simulink model "Op_Space_Grav_Comp"  (R2020b)
settings: Solver=VariableStepAuto  StartTime=0.0  StopTime=10  RelTol=1e-3
values from neighbouring files (symbols this model uses):
  G = myRobot.G_Lagrangian    [hw9_main.m]
  Ja = Ja(1:3,:)    [hw9_main.m]
  Kd = diag([25,15,15])    [hw9_main.m]
  Kp = diag([28,22,20])    [hw9_main.m]
  xd = [0.3; 0.3; 0.3]    [hw9_main.m]
settings Model: Creator=nicol  LastModifiedBy=nicol

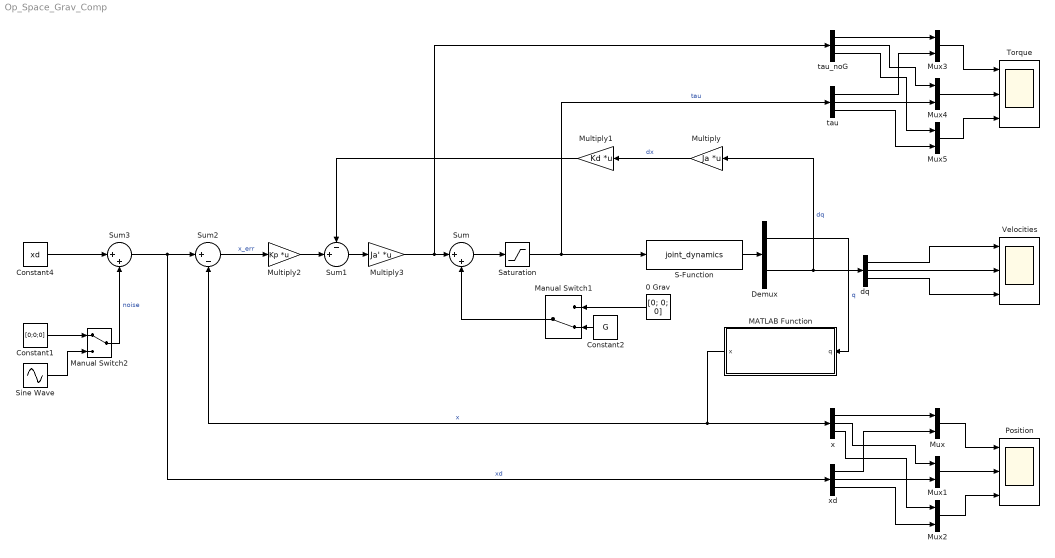
== system Op_Space_Grav_Comp ==
  0 Grav : Constant  Value=[0; 0; 0]  VectorParams1D=off
  Constant1 : Constant  Value=[0;0;0]  VectorParams1D=off
  Constant2 : Constant  Value=G  VectorParams1D=off
  Constant4 : Constant  Value=xd  VectorParams1D=off
  Demux : Demux  Outputs=2
  MATLAB Function : MATLAB Function  TreatAsAtomicUnit=on
  Manual Switch1 : ManualSwitch  CurrentSetting=0
  Manual Switch2 : ManualSwitch
  Multiply : Gain  Gain=Ja  Multiplication=Matrix(K*u)
  Multiply1 : Gain  Gain=Kd  Multiplication=Matrix(K*u)
  Multiply2 : Gain  Gain=Kp  Multiplication=Matrix(K*u)
  Multiply3 : Gain  Gain=Ja'  Multiplication=Matrix(K*u)
  Mux{,1..5} (6 alike) : Mux  Inputs=2
  Position : Scope  NumInputPorts=3
  S-Function : S-Function  FunctionName=joint_dynamics  Parameters=myRobot  SFunctionDeploymentMode=off  EnableBusSupport=off
  Saturation : Saturate  UpperLimit=50  LowerLimit=-50
  Sine Wave : Sin  Amplitude=0.1  SampleTime=0  VectorParams1D=off
  Sum : Sum  Inputs=|++
  Sum1 : Sum  Inputs=-+|
  Sum2 : Sum  Inputs=|+-
  Sum3 : Sum  Inputs=|++
  Torque : Scope  NumInputPorts=3
  Velocities : Scope  NumInputPorts=3
  dq : Demux  Outputs=3
  tau : Demux  Outputs=3
  tau_noG : Demux  Outputs=3
  x : Demux  Outputs=3
  xd : Demux  Outputs=3
  wires:
  Constant2/1 -> Manual Switch1/2
  Manual Switch1/1 -> Sum/2
  0 Grav/1 -> Manual Switch1/1
  Multiply1/1 -> Sum1/1
  Multiply2/1 -> Sum1/2
  Sum2/1 -> Multiply2/1  "x_err"
  Manual Switch2/1 -> Sum3/2  "noise"
  Constant1/1 -> Manual Switch2/1
  Sine Wave/1 -> Manual Switch2/2
  Constant4/1 -> Sum3/1
  Sum3/1 -> xd/1, Sum2/1  "xd"
  S-Function/1 -> Demux/1
  x/1 -> Mux/1
  xd/1 -> Mux/2
  x/2 -> Mux1/1
  xd/2 -> Mux1/2
  x/3 -> Mux2/1
  xd/3 -> Mux2/2
  Mux/1 -> Position/1
  Mux1/1 -> Position/2
  Mux2/1 -> Position/3
  dq/2 -> Velocities/2
  dq/1 -> Velocities/1
  dq/3 -> Velocities/3
  Demux/2 -> Multiply/1, dq/1  "dq"
  Saturation/1 -> S-Function/1, tau/1  "tau"
  Multiply/1 -> Multiply1/1  "dx"
  Sum1/1 -> Multiply3/1
  Multiply3/1 -> tau_noG/1, Sum/1
  Demux/1 -> MATLAB Function/1(q)  "q"
  MATLAB Function/1(x) -> x/1, Sum2/2  "x"
  Sum/1 -> Saturation/1
  tau/2 -> Mux4/2
  tau/3 -> Mux5/2
  Mux4/1 -> Torque/2
  Mux3/1 -> Torque/1
  Mux5/1 -> Torque/3
  tau_noG/1 -> Mux3/1
  tau_noG/2 -> Mux4/1
  tau/1 -> Mux3/2
  tau_noG/3 -> Mux5/1

== matlab function Op_Space_Grav_Comp/MATLAB Function ==
  data: q input size=3; x output size=3
function x = directKinematics(q)
x=[ q(1) + 1/5;
    q(3) + 1/5;
    q(2) + 1251/5000];
end
